simulink model "s_dbipridma"  (R2019b)
settings: Solver=ode1  StartTime=0.0  StopTime=100  FixedStep=0.001  RelTol=1e-3  EnableMultiTasking=on
values from neighbouring files (symbols this model uses):
  A = [0 0 1 0 ... (first row only)    [RIP_ABCD_SS.m]    (also in RIP_ABCD_SS_1.m; RIP_ABCD_SS_2.m = [0   0    1   0; RIP_ABCD_SS_3.m; RIP_ABCD_SS_POLE_PLACE.m)
  B = Kg * kt * B / Rm    [RIP_ABCD_SS.m]    (also in RIP_ABCD_SS_1.m; RIP_ABCD_SS_2.m; RIP_ABCD_SS_3.m; RIP_ABCD_SS_POLE_PLACE.m)
  C = eye(2,4)    [RIP_ABCD_SS.m]    (also in RIP_ABCD_SS_1.m; RIP_ABCD_SS_2.m = [1 0 0 0; RIP_ABCD_SS_3.m; RIP_ABCD_SS_POLE_PLACE.m)
  D = zeros(2,1)    [RIP_ABCD_SS.m]    (also in RIP_ABCD_SS_1.m; RIP_ABCD_SS_2.m = [0; RIP_ABCD_SS_3.m; RIP_ABCD_SS_POLE_PLACE.m)
  k = Kc*inv(W)    [RIP_ABCD_SS_POLE_PLACE.m]    (also in dripbalanced.m = lqr(Ai, Bi, Q, R))
  X0 = [-5, 1, -0.5, 0, 0, 0] * pi / 180    [dripbalanced.m]    (also in test_drip.m)
libraries: simulink_extras x5
settings Model: ExtModeTrigDuration=10000  ExtModeArmWhenConnect=off  Creator=MLevis  LastModifiedBy=Ridma
settings SolverCC: PositivePriorityOrder=on
settings DataIOCC: LimitDataPoints=on  SaveFormat=Array  SignalLoggingSaveFormat=ModelDataLogs  ReturnWorkspaceOutputs=off
settings OptimizationCC: BooleanDataType=off  OptimizeBlockIOStorage=off  BufferReuse=off  GlobalBufferReuse=off  ExpressionFolding=off  ExpressionDepthLimit=2147483647  LocalBlockOutputs=off  InitFltsAndDblsToZero=on  LifeSpan=inf  OptimizeDataStoreBuffers=off  BusAssignmentInplaceUpdate=off
settings DebuggingCC: SaveWithParameterizedLinksMsg=none  UnderspecifiedInitializationDetection=Classic  MergeDetectMultiDrivingBlocksExec=none  SignalResolutionControl=TryResolveAllWithWarning  MultiTaskDSMMsg=warning  MultiTaskCondExecSysMsg=none  FcnCallInpInsideContextMsg=warning  StateNameClashWarn=warning  SFUnexpectedBacktrackingDiag=warning  SFNoUnconditionalDefaultTransitionDiag=warning  SFExecutionAtInitializationDiag=none  ArithmeticOperatorsInVariantConditions=warning
settings HardwareCC: ProdBitPerPointer=32  ProdBitPerSizeT=32  ProdBitPerPtrDiffT=32  ProdLargestAtomicFloat=None  ProdIntDivRoundTo=Undefined  ProdEndianess=Unspecified  ProdWordSize=32  ProdHWDeviceType=32-bit Generic
settings ModelReferenceCC: PropagateSignalLabelsOutOfModel=off
settings SFSimCC: SimUseLocalCustomCode=off  CustomCodeUndefinedFunction=UseInterfaceOnly
settings RTWCC: Description=QuaRC Win32 Target  SystemTargetFile=quarc_windows.tlc  TemplateMakefile=quarc_default_tmf  RTWUseLocalCustomCode=off
settings CodeAppCC: StateflowObjectComments=on
settings STFCustomTargetCC: TargetFcnLib=ansi_tfl_tmw.mat  TargetPreCompLibLocation=C:\PROGRA~3\QUARC\lib\2011a\windows\release  GeneratePreprocessorConditionals=Disable all  CPPClassGenCompliant=on  GRTInterface=on  SystemTargetFile=quarc_windows.tlc
settings GRTTargetCC: TargetFcnLib=ansi_tfl_tmw.mat  TargetPreCompLibLocation=C:\PROGRA~3\QUARC\lib\2011a\windows\release  TargetLangStandard=C89/C90 (ANSI)  ParMdlRefBuildCompliant=off  CompOptLevelCompliant=off  ConcurrentExecutionCompliant=off  GeneratePreprocessorConditionals=Disable all  CombineOutputUpdateFcns=off  MatFileLogging=off  GRTInterface=on  UseToolchainInfoCompliant=off  ExtMode=on  ExtModeMexFile=quarc_comm
settings ConfigComp: CovMetricSettings=dw  CovHtmlReporting=on  CovSaveCumulativeToWorkspaceVar=on  CovSaveSingleToWorkspaceVar=on  CovExternalEMLEnable=off

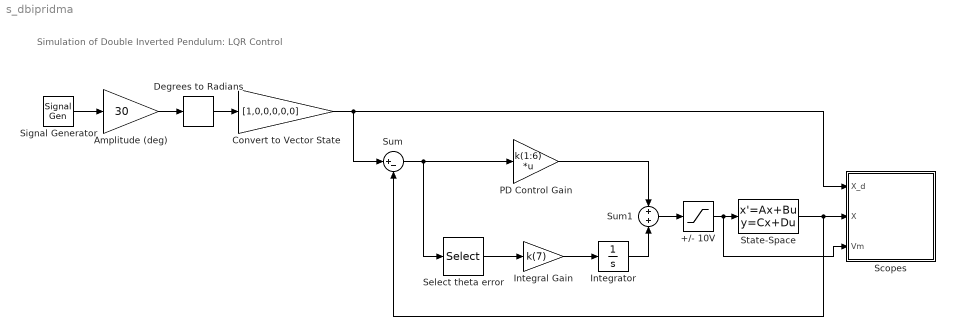
== system s_dbipridma ==
  note: Simulation of Double Inverted Pendulum: LQR Control
  +/- 10V : Saturate  UpperLimit=10  LowerLimit=-10
  Amplitude (deg) : Gain  Gain=30  SaturateOnIntegerOverflow=on  OutDataTypeStr=Inherit: Same as input  ParamDataTypeStr=Inherit: Same as input
  Convert to Vector State : Gain  Gain=[1,0,0,0,0,0]
  Degrees to Radians : simulink_extras/Transformations/Degrees to Radians
  Integral Gain : Gain  Gain=k(7)
  Integrator : Integrator
  PD Control Gain : Gain  Gain=k(1:6)  Multiplication=Matrix(K*u)  SaturateOnIntegerOverflow=on  OutDataTypeStr=Inherit: Same as input  ParamDataTypeStr=Inherit: Same as input
  Scopes : Subsystem
  Select theta error : Selector  InputPortWidth=6  IndexOptions=Index vector (dialog)  Indices=1  OutputSizes=1
  Signal Generator : SignalGenerator  WaveForm=square  Frequency=0.02
  State-Space : StateSpace  A=A  B=B  C=C  D=D  InitialCondition=X0
  Sum : Sum  Inputs=|+-
  Sum1 : Sum
  wires:
  Signal Generator/1 -> Amplitude (deg)/1
  Amplitude (deg)/1 -> Degrees to Radians/1
  Degrees to Radians/1 -> Convert to Vector State/1
  Convert to Vector State/1 -> Sum/1, Scopes/1(X_d)
  Sum/1 -> PD Control Gain/1, Select theta error/1
  Sum1/1 -> +/- 10V/1
  Integral Gain/1 -> Integrator/1
  Select theta error/1 -> Integral Gain/1
  Integrator/1 -> Sum1/2
  PD Control Gain/1 -> Sum1/1
  State-Space/1 -> Scopes/2(X), Sum/2
  +/- 10V/1 -> State-Space/1, Scopes/3(Vm)

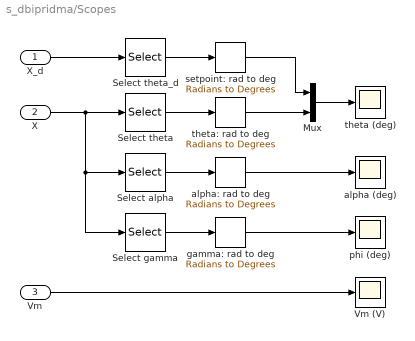
== system s_dbipridma/Scopes ==
  X_d : Inport
  X : Inport  Port=2
  Vm : Inport  Port=3
  Mux : Mux  Inputs=2
  Select alpha : Selector  InputPortWidth=6  IndexOptions=Index vector (dialog)  Indices=2  OutputSizes=1
  Select gamma : Selector  InputPortWidth=6  IndexOptions=Index vector (dialog)  Indices=3  OutputSizes=1
  Select theta : Selector  InputPortWidth=6  IndexOptions=Index vector (dialog)  Indices=1  OutputSizes=1
  Select theta_d : Selector  InputPortWidth=6  IndexOptions=Index vector (dialog)  Indices=1  OutputSizes=1
  Vm (V) : Scope
  alpha (deg) : Scope
  alpha: rad to deg : simulink_extras/Transformations/Radians to Degrees
  gamma: rad to deg : simulink_extras/Transformations/Radians to Degrees
  phi (deg) : Scope
  setpoint: rad to deg : simulink_extras/Transformations/Radians to Degrees
  theta (deg) : Scope
  theta: rad to deg : simulink_extras/Transformations/Radians to Degrees
  wires:
  X/1 -> Select theta/1, Select alpha/1, Select gamma/1
  alpha: rad to deg/1 -> alpha (deg)/1
  gamma: rad to deg/1 -> phi (deg)/1
  Select theta/1 -> theta: rad to deg/1
  Select alpha/1 -> alpha: rad to deg/1
  Select gamma/1 -> gamma: rad to deg/1
  theta: rad to deg/1 -> Mux/2
  Mux/1 -> theta (deg)/1
  X_d/1 -> Select theta_d/1
  setpoint: rad to deg/1 -> Mux/1
  Select theta_d/1 -> setpoint: rad to deg/1
  Vm/1 -> Vm (V)/1
